simulink model "airbrakes"  (R2025b)
settings: Solver=VariableStepAuto  StartTime=0.0  StopTime=20  RelTol=1e-3
settings Model: Creator=2015k  LastModifiedBy=2015k

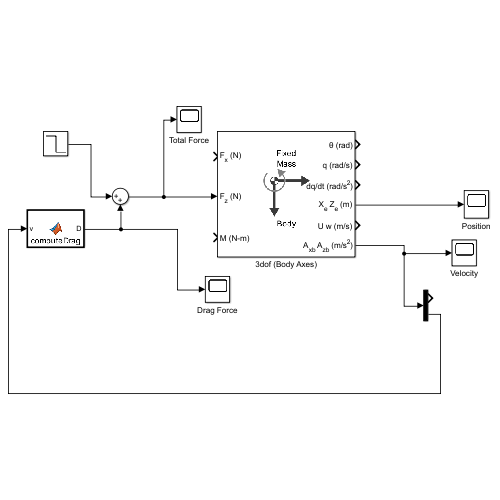
[thumbnail: Simulink's stored preview of the top-level diagram]
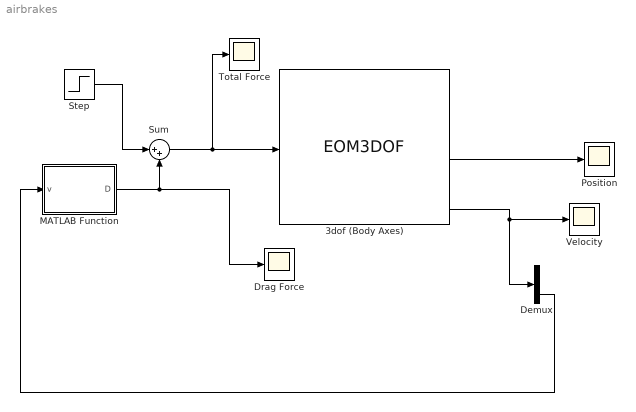
== system airbrakes ==
  3dof (Body Axes) : EOM3DOF  v_ini=0  g=-9.81
  Demux : Demux  Outputs=2
  Drag Force : Scope
      settings: DataLoggingVariableName=ScopeData2
  MATLAB Function : MATLAB Function  TreatAsAtomicUnit=on
  Position : Scope
      settings: ActiveDisplayYMinimum=-31.049999999999994  ActiveDisplayYMaximum=279.45
  Step : Step  Time=1.8  Before=44  After=0  SampleTime=0
  Sum : Sum  Inputs=|++
  Total Force : Scope
      settings: DataLoggingVariableName=ScopeData3
  Velocity : Scope
      settings: ActiveDisplayYMinimum=-15.309999999999999  ActiveDisplayYMaximum=39.69
  wires:
  3dof (Body Axes)/4 -> Position/1
  3dof (Body Axes)/6 -> Demux/1, Velocity/1
  Step/1 -> Sum/1
  MATLAB Function/1(D) -> Drag Force/1, Sum/2
  Sum/1 -> Total Force/1, 3dof (Body Axes)/2
  Demux/2 -> MATLAB Function/1(v)

== matlab function airbrakes/MATLAB Function ==
  data: v input; D output
function D = computeDrag(v)

% A - Rocket Reference Area (cross sectional area)
% v - Current Velocity
% rho - Atmospheric Density
% C_D - Drag Coefficient

A = 0.00353; % m^2 - get right units
rho = 1.44; % kg/m^3
C_D = 0.4;

% Negative sign for drag to be applied towards ground direction
D = -0.5 * C_D * rho * A * (v^2);

end
